simulink model "model"  (R2016a)
settings: Solver=FixedStepAuto  SolverMode=SingleTasking  StartTime=0.0  StopTime=160  FixedStep=0.001  RelTol=1e-3
values from neighbouring files (symbols this model uses):
  counting_treshold = 1    [variablen.m]
  lower_limit = 0.1    [variablen.m]
  time_exceed = 20    [variablen.m]
  tooth_ratio = 44/counting_treshold    (= 44)    [variablen.m]
  upper_limit = 0.8    [variablen.m]
  wheel_circumference = 1.83    [variablen.m]
libraries: simulink x5
settings Model: Creator=frede  LastModifiedBy=frede
settings DebuggingCC: SFUnexpectedBacktrackingDiag=error  SFNoUnconditionalDefaultTransitionDiag=error
settings GRTTargetCC: TargetLangStandard=C99 (ISO)  GeneratePreprocessorConditionals=Use local settings
settings ConfigComp: CovMetricSettings=dwe  CovHtmlReporting=off  CovSaveCumulativeToWorkspaceVar=off  CovSaveSingleToWorkspaceVar=off  CovExternalEMLEnable=on

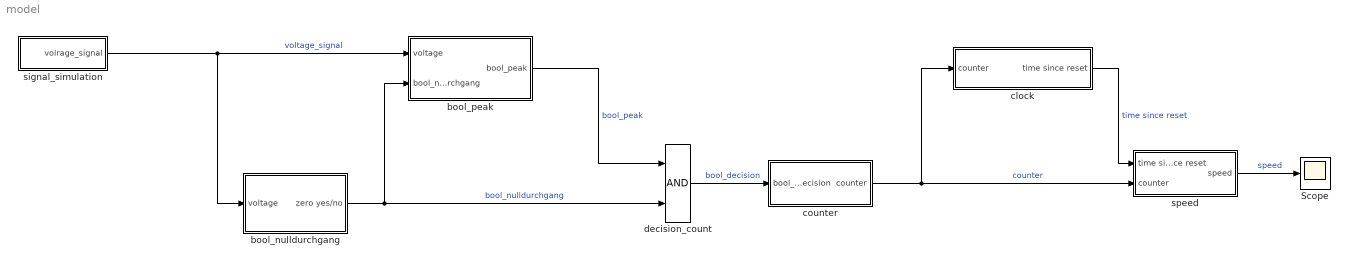
== system model ==
  Scope : Scope
  "bool_nulldurchgang " : Subsystem
  bool_peak : Subsystem
  clock : Subsystem
  counter : Subsystem
  decision_count : Logic  AllPortsSameDT=off  OutDataTypeStr=boolean
  signal_simulation : Subsystem
  speed : Subsystem
  wires:
  "bool_nulldurchgang "/1(zero yes/no) -> decision_count/2, bool_peak/2(bool_nulldurchgang)  "bool_nulldurchgang"
  bool_peak/1(bool_peak) -> decision_count/1  "bool_peak"
  decision_count/1 -> counter/1(bool_decision)  "bool_decision"
  clock/1(time since reset) -> speed/1(time since reset)  "time since reset"
  counter/1(counter) -> speed/2(counter), clock/1(counter)  "counter"
  speed/1(speed) -> Scope/1  "speed"
  signal_simulation/1(volrage_signal) -> bool_peak/1(voltage), "bool_nulldurchgang "/1(voltage)  "voltage_signal"

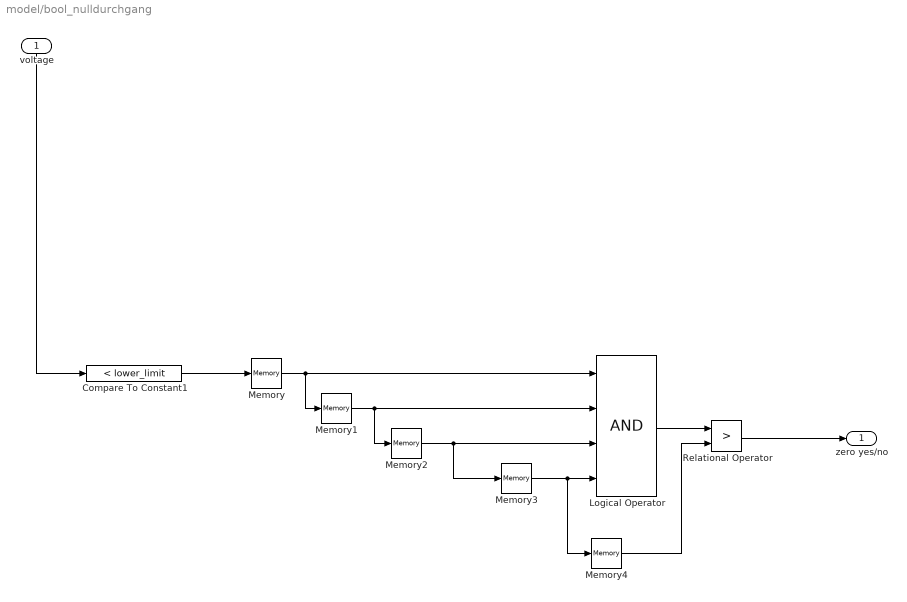
== system model/bool_nulldurchgang  ==
  voltage : Inport
  Compare To Constant1 : simulink/Logic and Bit Operations/Compare To Constant  relop=<  const=lower_limit  OutDataTypeStr=boolean
  Logical Operator : Logic  Inputs=4  AllPortsSameDT=off  OutDataTypeStr=boolean
  Memory{,1..4} (5 alike) : Memory
  Relational Operator : RelationalOperator  Operator=>  OutDataTypeStr=boolean
  zero yes/no : Outport
  wires:
  Relational Operator/1 -> zero yes/no/1
  Logical Operator/1 -> Relational Operator/1
  Memory2/1 -> Memory3/1, Logical Operator/3
  Memory1/1 -> Memory2/1, Logical Operator/2
  Memory/1 -> Logical Operator/1, Memory1/1
  Memory4/1 -> Relational Operator/2
  Memory3/1 -> Logical Operator/4, Memory4/1
  Compare To Constant1/1 -> Memory/1
  voltage/1 -> Compare To Constant1/1

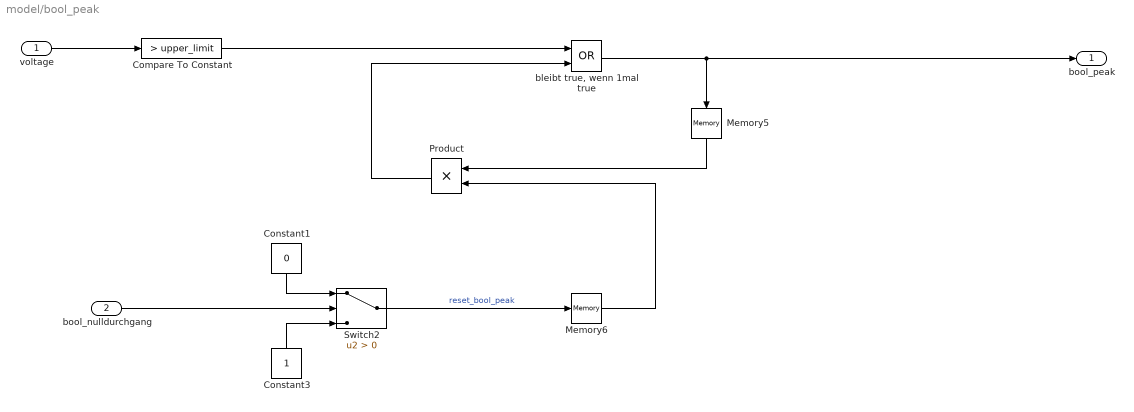
== system model/bool_peak ==
  voltage : Inport
  bool_nulldurchgang : Inport  Port=2
  Compare To Constant : simulink/Logic and Bit Operations/Compare To Constant  relop=>  const=upper_limit  OutDataTypeStr=boolean
  Constant1 : Constant  Value=0
  Constant3 : Constant
  Memory5 : Memory
  Memory6 : Memory
  Product : Product
  Switch2 : Switch  Criteria=u2 > Threshold
  "bleibt true, wenn 1mal true" : Logic  Operator=OR  AllPortsSameDT=off  OutDataTypeStr=boolean
  bool_peak : Outport
  wires:
  voltage/1 -> Compare To Constant/1
  Product/1 -> "bleibt true, wenn 1mal true"/2
  Memory6/1 -> Product/2
  "bleibt true, wenn 1mal true"/1 -> bool_peak/1, Memory5/1
  Constant3/1 -> Switch2/3
  bool_nulldurchgang/1 -> Switch2/2
  Constant1/1 -> Switch2/1
  Switch2/1 -> Memory6/1  "reset_bool_peak"
  Memory5/1 -> Product/1
  Compare To Constant/1 -> "bleibt true, wenn 1mal true"/1

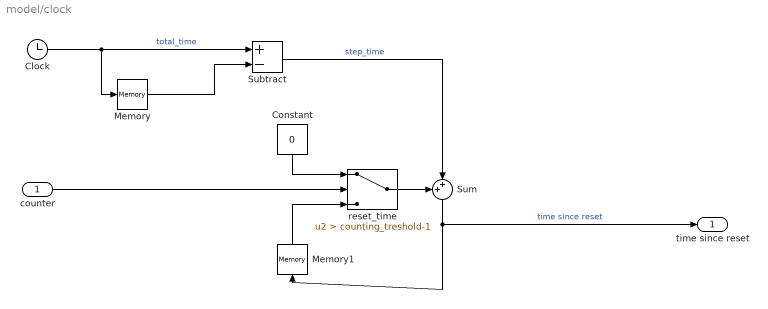
== system model/clock ==
  counter : Inport
  Clock : Clock
  Constant : Constant  Value=0
  Memory : Memory
  Memory1 : Memory
  Subtract : Sum  Inputs=+-
  Sum : Sum  Inputs=++|
  reset_time : Switch  Criteria=u2 > Threshold  Threshold=counting_treshold-1
  time since reset : Outport
  wires:
  Clock/1 -> Subtract/1, Memory/1  "total_time"
  Memory/1 -> Subtract/2
  Subtract/1 -> Sum/2  "step_time"
  Sum/1 -> time since reset/1, Memory1/1  "time since reset"
  counter/1 -> reset_time/2
  Memory1/1 -> reset_time/3
  reset_time/1 -> Sum/1
  Constant/1 -> reset_time/1

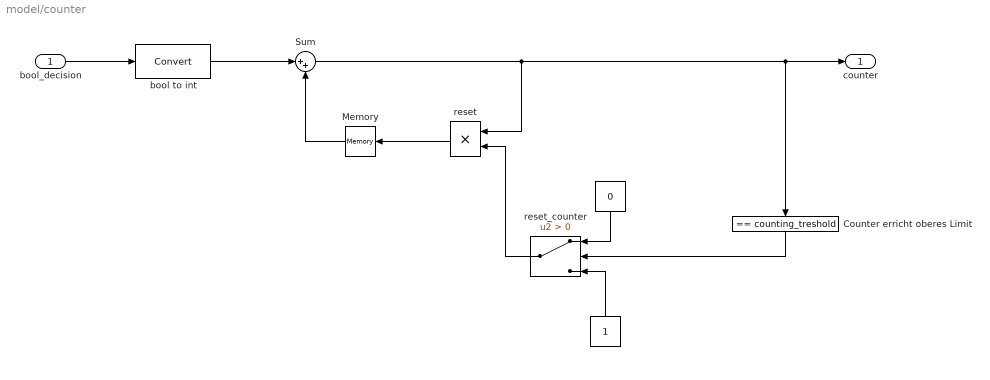
== system model/counter ==
  bool_decision : Inport
  "  " : Constant
  "   " : Constant  Value=0
  Counter erricht oberes Limit : simulink/Logic and Bit Operations/Compare To Constant  relop===  const=counting_treshold  OutDataTypeStr=boolean
  Memory : Memory
  Sum : Sum  Inputs=|++
  bool to int : DataTypeConversion  OutMin=1
  reset : Product
  reset_counter : Switch  Criteria=u2 > Threshold
  counter : Outport
  wires:
  bool_decision/1 -> bool to int/1
  Memory/1 -> Sum/2
  reset/1 -> Memory/1
  reset_counter/1 -> reset/2
  bool to int/1 -> Sum/1
  Sum/1 -> counter/1, Counter erricht oberes Limit/1, reset/1
  Counter erricht oberes Limit/1 -> reset_counter/2
  "  "/1 -> reset_counter/3
  "   "/1 -> reset_counter/1

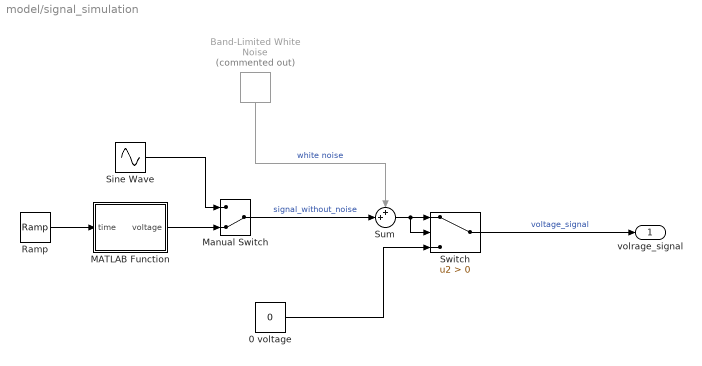
== system model/signal_simulation ==
  0 voltage : Constant  Value=0
  Band-Limited White Noise : simulink/Sources/Band-Limited White Noise  Commented=on  Cov=0.001  Ts=0.1  seed=[23341]
  MATLAB Function : MATLAB Function  TreatAsAtomicUnit=on
  Manual Switch : ManualSwitch  CurrentSetting=0
  Ramp : simulink/Sources/Ramp  slope=1  start=0  X0=0
  Sine Wave : Sin  Frequency=10  SampleTime=0
  Sum : Sum  Inputs=++|
  Switch : Switch  Criteria=u2 > Threshold
  volrage_signal : Outport
  wires:
  Sum/1 -> Switch/2, Switch/1
  Manual Switch/1 -> Sum/2  "signal_without_noise"
  0 voltage/1 -> Switch/3
  Ramp/1 -> MATLAB Function/1(time)
  Sine Wave/1 -> Manual Switch/1
  MATLAB Function/1(voltage) -> Manual Switch/2
  Switch/1 -> volrage_signal/1  "voltage_signal"
  Band-Limited White Noise/1 -> Sum/1  "white noise"

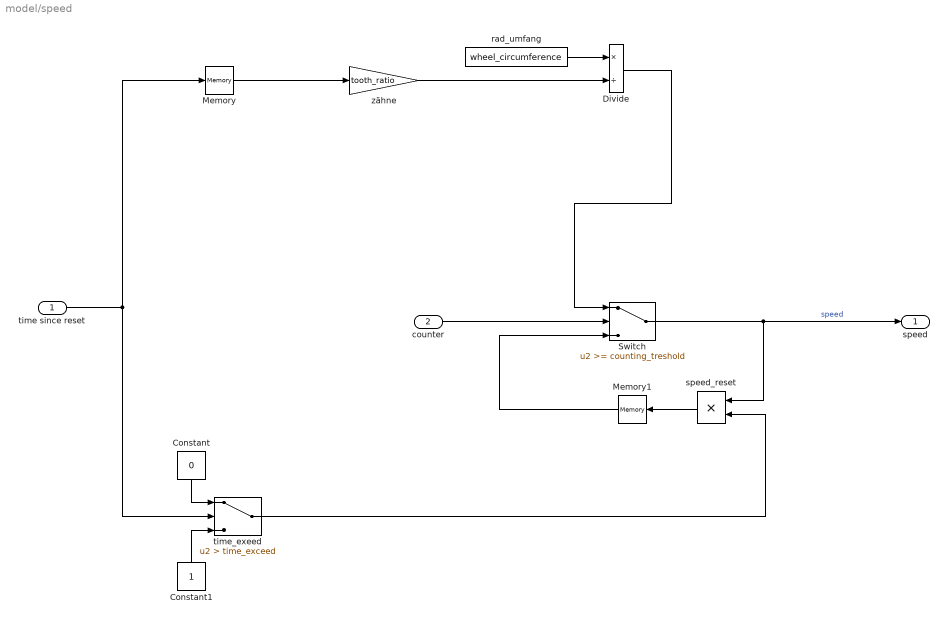
== system model/speed ==
  time since reset : Inport
  counter : Inport  Port=2
  Constant : Constant  Value=0
  Constant1 : Constant
  Divide : Product  Inputs=*/
  Memory : Memory
  Memory1 : Memory
  Switch : Switch  Threshold=counting_treshold
  rad_umfang : Constant  Value=wheel_circumference
  speed_reset : Product
  time_exeed : Switch  Criteria=u2 > Threshold  Threshold=time_exceed
  zähne : Gain  Gain=tooth_ratio
  speed : Outport
  wires:
  time since reset/1 -> Memory/1, time_exeed/2
  rad_umfang/1 -> Divide/1
  Divide/1 -> Switch/1
  zähne/1 -> Divide/2
  counter/1 -> Switch/2
  Switch/1 -> speed_reset/1, speed/1  "speed"
  Memory1/1 -> Switch/3
  Constant1/1 -> time_exeed/3
  Constant/1 -> time_exeed/1
  speed_reset/1 -> Memory1/1
  time_exeed/1 -> speed_reset/2
  Memory/1 -> zähne/1

== matlab function model/signal_simulation/MATLAB Function ==
  data: time input; voltage output
function voltage = fcn(time)
if (time < 40 )
    voltage=sin(time);
elseif time < 80
voltage=sin(5*time);
 
else 
    voltage =0;
end
